simulink model "example2"  (R2022a)
settings: Solver=FixedStepAuto  StartTime=0.0  StopTime=20  FixedStep=0.01  RelTol=1e-3
values from neighbouring files (symbols this model uses):
  i0 = x0(i,1)    [gen_data.m]
  v0 = x0(i,2)    [gen_data.m]
settings Model: Creator=diego  LastModifiedBy=diego

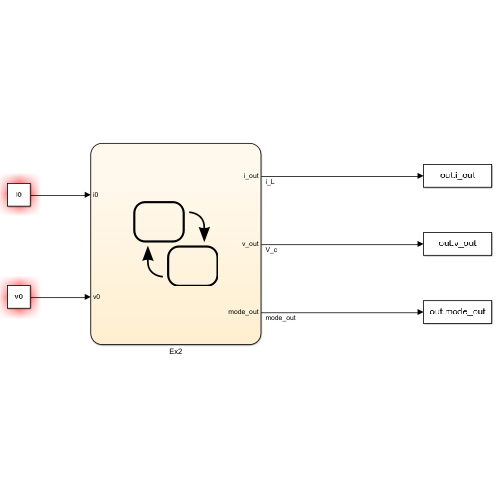
[thumbnail: Simulink's stored preview of the top-level diagram]
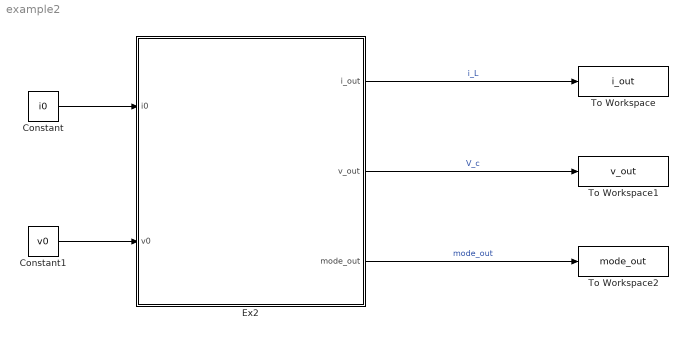
== system example2 ==
  Constant : Constant  Value=i0
  Constant1 : Constant  Value=v0
  Ex2 : Stateflow chart  TreatAsAtomicUnit=on
  To Workspace : ToWorkspace  VariableName=i_out  SampleTime=-1
  To Workspace1 : ToWorkspace  VariableName=v_out  SampleTime=-1
  To Workspace2 : ToWorkspace  VariableName=mode_out  SampleTime=-1
  wires:
  Constant/1 -> Ex2/1(i0)
  Constant1/1 -> Ex2/2(v0)
  Ex2/1(i_out) -> To Workspace/1  "i_L"
  Ex2/3(mode_out) -> To Workspace2/1  "mode_out"
  Ex2/2(v_out) -> To Workspace1/1  "V_c"

== stateflow chart example2/Ex2 ==
  settings: updateMethod=CONTINUOUS
  state Mode1
    du:
    i_dot = 1;
    v_dot = i;
    t_dot = 1;
    i_out = i;
    v_out = v;
    mode_out=1;
  state Mode2
    du:
    i_dot = -v^2;
    v_dot = -1;
    t_dot = 1;
    i_out = i;
    v_out = v;
    mode_out=2;
  Mode2 -> Mode1 : [v < 0]
  Mode1 -> Mode2 : [i > 2]
  (default) -> Mode1 : {i = i0;
      | v = v0;}
  data: t local double; i_out output double; v_out output double; i local double; v local double; i0 input double; v0 input double; mode_out output double
  data t settings: updateMethod=SF_CONTINUOUS_TIME_DATA
  data i settings: updateMethod=SF_CONTINUOUS_TIME_DATA
  data v settings: updateMethod=SF_CONTINUOUS_TIME_DATA
